simulink model "btms_csi_ebc"  (R2025a)
settings: Solver=VariableStepAuto  StartTime=0.0  StopTime=10.0  RelTol=1e-3
settings Model: Creator=adam  LastModifiedBy=adam

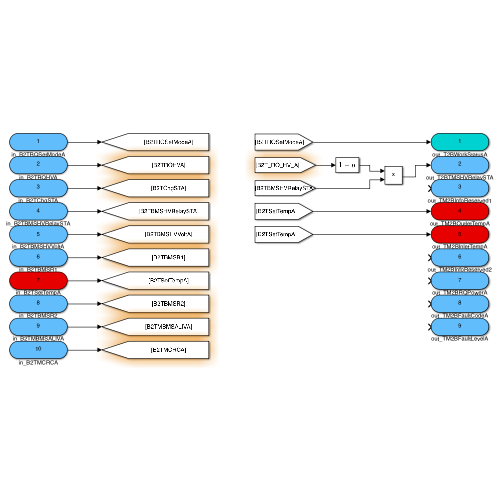
[thumbnail: Simulink's stored preview of the top-level diagram]
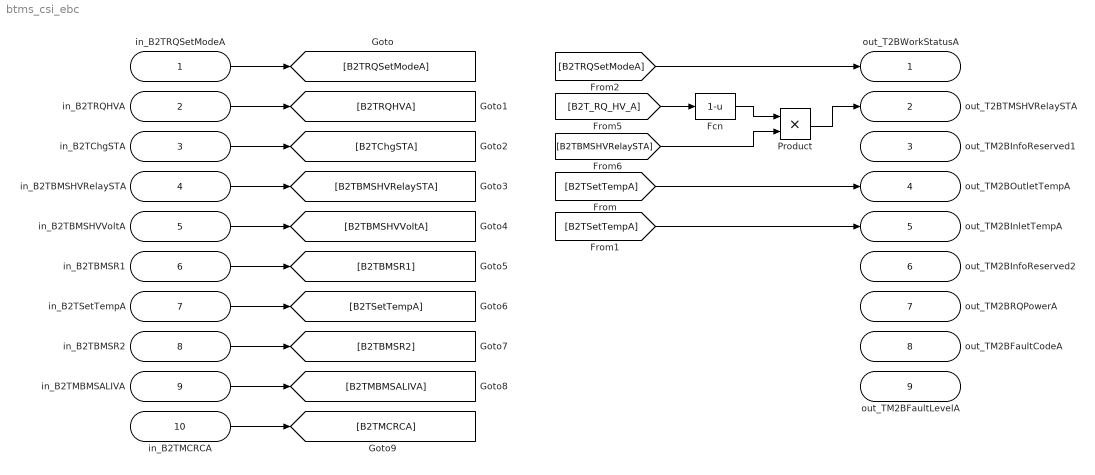
== system btms_csi_ebc ==
  in_B2TRQSetModeA : Inport
  in_B2TRQHVA : Inport  Port=2
  in_B2TChgSTA : Inport  Port=3
  in_B2TBMSHVRelaySTA : Inport  Port=4
  in_B2TBMSHVVoltA : Inport  Port=5
  in_B2TBMSR1 : Inport  Port=6
  in_B2TSetTempA : Inport  Port=7
  in_B2TBMSR2 : Inport  Port=8
  in_B2TMBMSALIVA : Inport  Port=9
  in_B2TMCRCA : Inport  Port=10
  Fcn : Fcn  Expr=1-u
  Product : Product
  out_T2BWorkStatusA : Outport
  out_T2BTMSHVRelaySTA : Outport  Port=2
  out_TM2BInfoReserved1 : Outport  Port=3
  out_TM2BOutletTempA : Outport  Port=4
  out_TM2BInletTempA : Outport  Port=5
  out_TM2BInfoReserved2 : Outport  Port=6
  out_TM2BRQPowerA : Outport  Port=7
  out_TM2BFaultCodeA : Outport  Port=8
  out_TM2BFaultLevelA : Outport  Port=9
  wires:
  [B2TRQSetModeA] -> out_T2BWorkStatusA/1
  [B2TSetTempA] -> out_TM2BOutletTempA/1
  [B2TSetTempA] -> out_TM2BInletTempA/1
  in_B2TRQSetModeA/1 -> [B2TRQSetModeA]
  in_B2TRQHVA/1 -> [B2TRQHVA]
  in_B2TChgSTA/1 -> [B2TChgSTA]
  in_B2TBMSHVRelaySTA/1 -> [B2TBMSHVRelaySTA]
  in_B2TBMSHVVoltA/1 -> [B2TBMSHVVoltA]
  in_B2TBMSR1/1 -> [B2TBMSR1]
  in_B2TSetTempA/1 -> [B2TSetTempA]
  in_B2TBMSR2/1 -> [B2TBMSR2]
  in_B2TMBMSALIVA/1 -> [B2TMBMSALIVA]
  in_B2TMCRCA/1 -> [B2TMCRCA]
  Fcn/1 -> Product/1
  [B2TBMSHVRelaySTA] -> Product/2
  [B2T_RQ_HV_A] -> Fcn/1
  Product/1 -> out_T2BTMSHVRelaySTA/1
